simulink model "MotorDriveThermalTestbench"  (R2024b)
settings: Solver=daessc  StartTime=0.0  StopTime=2400  FixedStep=dt  RelTol=1e-3  AbsTol=1e-3
PreLoadFcn:
  | % Simulation parameters
  | MotorDriveThermalTestBenchParams;
model workspace (MAT data in the model file):
  V_frac_bridge = 0.0437
  V_fract_teeth = 0.9563
values from neighbouring files (symbols this model uses):
  CaseParams = struct()    [InverterThermalParams.m]
  HeatsinkParams = struct()    [InverterThermalParams.m]
undefined symbols (not defined in the file or in its folder): electricDrive, H_AH, H_AL, H_BH, H_BL, H_CH, H_CL, PipeParams, vehicleThermal
libraries: fl_lib x171, ee_lib x31, nesl_utility x28, nesl_utility_internal x12, sdl_lib x6, SimscapeFluids_lib x3, autolibshared x1
(part 4 of 4)

== system MotorDriveThermalTestbench/Motor Cooling/windingOilJet/ThermalResistance /Oil Wet Area ==
  PS Divide : fl_lib/Physical Signals/Functions/PS Divide
  PS Gain : fl_lib/Physical Signals/Functions/PS Gain  gain=pi
  PS Product : fl_lib/Physical Signals/Functions/PS Product
  PS Product1 : fl_lib/Physical Signals/Functions/PS Product
  Q : PMIOPort  Side=Left
  oilThickness : PMIOPort  Port=2  Side=Left
  v : PMIOPort  Port=3  Side=Left
  OD : PMIOPort  Port=4  Side=Left
  Area : PMIOPort  Port=5  Side=Right
  connections:
  Q/RConn1 -- PS Divide/LConn1
  v/RConn1 -- PS Product/LConn2
  oilThickness/RConn1 -- PS Product/LConn1
  PS Product1/RConn1 -- Area/RConn1
  PS Gain/RConn1 -- PS Product1/LConn2
  PS Product/RConn1 -- PS Divide/LConn2
  PS Divide/RConn1 -- PS Product1/LConn1
  OD/RConn1 -- PS Gain/LConn1

== system MotorDriveThermalTestbench/Motor Cooling/windingOilJet/ThermalResistance /ReynoldsNo ==
  KinamaticVisc : fl_lib/Physical Signals/Sources/PS Constant  constant=electricDrive.MotorThermal.KinVisc*1e-6 m^2/s
  PS Divide : fl_lib/Physical Signals/Functions/PS Divide
  PS Gain : fl_lib/Physical Signals/Functions/PS Gain  gain=pi
  PS Product : fl_lib/Physical Signals/Functions/PS Product
  v : PMIOPort  Side=Left
  od : PMIOPort  Port=2  Side=Left
  Re : PMIOPort  Port=3  Side=Right
  connections:
  KinamaticVisc/RConn1 -- PS Divide/LConn2
  od/RConn1 -- PS Gain/LConn1
  PS Gain/RConn1 -- PS Product/LConn2
  PS Product/RConn1 -- PS Divide/LConn1
  PS Divide/RConn1 -- Re/RConn1
  v/RConn1 -- PS Product/LConn1

== system MotorDriveThermalTestbench/Motor Cooling/windingOilJet/ThermalResistance /avgDriftVelocity ==
  "Jet Velocity " : fl_lib/Physical Signals/Sources/PS Constant  constant=0.5 m/s
  PS Add : fl_lib/Physical Signals/Functions/PS Add
  PS Add1 : fl_lib/Physical Signals/Functions/PS Add
  PS Gain : fl_lib/Physical Signals/Functions/PS Gain  gain=2*9.81 m/s^2
  PS Gain1 : fl_lib/Physical Signals/Functions/PS Gain  gain=0.5
  PS Math Function : fl_lib/Physical Signals/Functions/PS Math Function  fcn_choice=foundation.enum.math_function.square  v=1
  PS Math Function1 : fl_lib/Physical Signals/Functions/PS Math Function  fcn_choice=foundation.enum.math_function.sqrt  v=1
  vd : PMIOPort  Side=Right
  v : PMIOPort  Port=2  Side=Left
  connections:
  PS Gain/RConn1 -- PS Add/LConn2
  PS Math Function/RConn1 -- PS Add/LConn1
  PS Math Function1/RConn1 -- PS Add1/LConn2
  v/RConn1 -- PS Gain/LConn1
  "Jet Velocity "/RConn1 -- PS Math Function/LConn1 -- PS Add1/LConn1
  PS Add/RConn1 -- PS Math Function1/LConn1
  PS Gain1/LConn1 -- PS Add1/RConn1
  PS Gain1/RConn1 -- vd/RConn1

== system MotorDriveThermalTestbench/Test Env N Controls/Motor speed N test environment/Test Environment/Setting ==
  note: Road Wind & Brake
  dec : Inport
  Brake : Constant  Value=0
  Brake1 : Constant
  Bus : Subsystem
  Road Inclination : Constant  Value=0
  Switch : Switch  Criteria=u2 > Threshold  Threshold=-20.557  SaturateOnIntegerOverflow=off  InputSameDT=off
  Wind Speed : Constant  Value=0
  b : Outport
  wires:
  Bus/1(b) -> b/1
  Brake1/1 -> Switch/3
  Brake/1 -> Switch/1
  Switch/1 -> Bus/3(Br)
  dec/1 -> Switch/2
  Road Inclination/1 -> Bus/1(In)
  Wind Speed/1 -> Bus/2(Wi)

== system MotorDriveThermalTestbench/Inverter/DetailedInverter/BaseplateAndHeatsink/BasePLT/meas_AH ==
  Heat Flow Rate Sensor : fl_lib/Thermal/Thermal Sensors/Heat Flow Rate Sensor
  PS-Simulink Converter : nesl_utility_internal/PS-Simulink Converter  PhysicalDomain=network_engine_domain  SubClassName=ps_output  LeftPortType=input  RightPortType=output  PseudoPeriodic=off  Frequencies=[]  VectorFormat=inherit  Unit=degC  AffineConversion=on
  PS-Simulink Converter1 : nesl_utility_internal/PS-Simulink Converter  PhysicalDomain=network_engine_domain  SubClassName=ps_output  LeftPortType=input  RightPortType=output  PseudoPeriodic=off  Frequencies=[]  VectorFormat=inherit  Unit=W  AffineConversion=off
  Temperature Sensor : fl_lib/Thermal/Thermal Sensors/Temperature Sensor  temperature_measure=foundation.enum.MeasurementReference.difference
  Thermal Reference : fl_lib/Thermal/Thermal Elements/Thermal Reference
  A : PMIOPort  Side=Left
  B : PMIOPort  Port=2  Side=Right
  T : Outport
  Q : Outport  Port=2
  wires:
  PS-Simulink Converter/1 -> T/1
  PS-Simulink Converter1/1 -> Q/1
  connections:
  Temperature Sensor/LConn1 -- A/RConn1 -- Heat Flow Rate Sensor/LConn1
  Thermal Reference/LConn1 -- Temperature Sensor/RConn1
  PS-Simulink Converter/LConn1 -- Temperature Sensor/RConn2
  B/RConn1 -- Heat Flow Rate Sensor/RConn2
  Heat Flow Rate Sensor/RConn1 -- PS-Simulink Converter1/LConn1

== system MotorDriveThermalTestbench/Inverter/DetailedInverter/BaseplateAndHeatsink/BasePLT/meas_AL ==
  Heat Flow Rate Sensor : fl_lib/Thermal/Thermal Sensors/Heat Flow Rate Sensor
  PS-Simulink Converter : nesl_utility_internal/PS-Simulink Converter  PhysicalDomain=network_engine_domain  SubClassName=ps_output  LeftPortType=input  RightPortType=output  PseudoPeriodic=off  Frequencies=[]  VectorFormat=inherit  Unit=degC  AffineConversion=on
  PS-Simulink Converter1 : nesl_utility_internal/PS-Simulink Converter  PhysicalDomain=network_engine_domain  SubClassName=ps_output  LeftPortType=input  RightPortType=output  PseudoPeriodic=off  Frequencies=[]  VectorFormat=inherit  Unit=W  AffineConversion=off
  Temperature Sensor : fl_lib/Thermal/Thermal Sensors/Temperature Sensor  temperature_measure=foundation.enum.MeasurementReference.difference
  Thermal Reference : fl_lib/Thermal/Thermal Elements/Thermal Reference
  A : PMIOPort  Side=Left
  B : PMIOPort  Port=2  Side=Right
  T : Outport
  Q : Outport  Port=2
  wires:
  PS-Simulink Converter/1 -> T/1
  PS-Simulink Converter1/1 -> Q/1
  connections:
  Heat Flow Rate Sensor/LConn1 -- Temperature Sensor/LConn1 -- A/RConn1
  Thermal Reference/LConn1 -- Temperature Sensor/RConn1
  PS-Simulink Converter/LConn1 -- Temperature Sensor/RConn2
  B/RConn1 -- Heat Flow Rate Sensor/RConn2
  Heat Flow Rate Sensor/RConn1 -- PS-Simulink Converter1/LConn1

== system MotorDriveThermalTestbench/Inverter/DetailedInverter/BaseplateAndHeatsink/BasePLT/meas_BH ==
  Heat Flow Rate Sensor : fl_lib/Thermal/Thermal Sensors/Heat Flow Rate Sensor
  PS-Simulink Converter : nesl_utility_internal/PS-Simulink Converter  PhysicalDomain=network_engine_domain  SubClassName=ps_output  LeftPortType=input  RightPortType=output  PseudoPeriodic=off  Frequencies=[]  VectorFormat=inherit  Unit=degC  AffineConversion=on
  PS-Simulink Converter1 : nesl_utility_internal/PS-Simulink Converter  PhysicalDomain=network_engine_domain  SubClassName=ps_output  LeftPortType=input  RightPortType=output  PseudoPeriodic=off  Frequencies=[]  VectorFormat=inherit  Unit=W  AffineConversion=off
  Temperature Sensor : fl_lib/Thermal/Thermal Sensors/Temperature Sensor  temperature_measure=foundation.enum.MeasurementReference.difference
  Thermal Reference : fl_lib/Thermal/Thermal Elements/Thermal Reference
  A : PMIOPort  Side=Left
  B : PMIOPort  Port=2  Side=Right
  T : Outport
  Q : Outport  Port=2
  wires:
  PS-Simulink Converter/1 -> T/1
  PS-Simulink Converter1/1 -> Q/1
  connections:
  Heat Flow Rate Sensor/LConn1 -- Temperature Sensor/LConn1 -- A/RConn1
  Thermal Reference/LConn1 -- Temperature Sensor/RConn1
  PS-Simulink Converter/LConn1 -- Temperature Sensor/RConn2
  B/RConn1 -- Heat Flow Rate Sensor/RConn2
  Heat Flow Rate Sensor/RConn1 -- PS-Simulink Converter1/LConn1

== system MotorDriveThermalTestbench/Inverter/DetailedInverter/BaseplateAndHeatsink/BasePLT/meas_BL ==
  Heat Flow Rate Sensor : fl_lib/Thermal/Thermal Sensors/Heat Flow Rate Sensor
  PS-Simulink Converter : nesl_utility_internal/PS-Simulink Converter  PhysicalDomain=network_engine_domain  SubClassName=ps_output  LeftPortType=input  RightPortType=output  PseudoPeriodic=off  Frequencies=[]  VectorFormat=inherit  Unit=degC  AffineConversion=on
  PS-Simulink Converter1 : nesl_utility_internal/PS-Simulink Converter  PhysicalDomain=network_engine_domain  SubClassName=ps_output  LeftPortType=input  RightPortType=output  PseudoPeriodic=off  Frequencies=[]  VectorFormat=inherit  Unit=W  AffineConversion=off
  Temperature Sensor : fl_lib/Thermal/Thermal Sensors/Temperature Sensor  temperature_measure=foundation.enum.MeasurementReference.difference
  Thermal Reference : fl_lib/Thermal/Thermal Elements/Thermal Reference
  A : PMIOPort  Side=Left
  B : PMIOPort  Port=2  Side=Right
  T : Outport
  Q : Outport  Port=2
  wires:
  PS-Simulink Converter/1 -> T/1
  PS-Simulink Converter1/1 -> Q/1
  connections:
  Heat Flow Rate Sensor/LConn1 -- Temperature Sensor/LConn1 -- A/RConn1
  Thermal Reference/LConn1 -- Temperature Sensor/RConn1
  PS-Simulink Converter/LConn1 -- Temperature Sensor/RConn2
  B/RConn1 -- Heat Flow Rate Sensor/RConn2
  Heat Flow Rate Sensor/RConn1 -- PS-Simulink Converter1/LConn1

== system MotorDriveThermalTestbench/Inverter/DetailedInverter/BaseplateAndHeatsink/BasePLT/meas_CH ==
  Heat Flow Rate Sensor : fl_lib/Thermal/Thermal Sensors/Heat Flow Rate Sensor
  PS-Simulink Converter : nesl_utility_internal/PS-Simulink Converter  PhysicalDomain=network_engine_domain  SubClassName=ps_output  LeftPortType=input  RightPortType=output  PseudoPeriodic=off  Frequencies=[]  VectorFormat=inherit  Unit=degC  AffineConversion=on
  PS-Simulink Converter1 : nesl_utility_internal/PS-Simulink Converter  PhysicalDomain=network_engine_domain  SubClassName=ps_output  LeftPortType=input  RightPortType=output  PseudoPeriodic=off  Frequencies=[]  VectorFormat=inherit  Unit=W  AffineConversion=off
  Temperature Sensor : fl_lib/Thermal/Thermal Sensors/Temperature Sensor  temperature_measure=foundation.enum.MeasurementReference.difference
  Thermal Reference : fl_lib/Thermal/Thermal Elements/Thermal Reference
  A : PMIOPort  Side=Left
  B : PMIOPort  Port=2  Side=Right
  T : Outport
  Q : Outport  Port=2
  wires:
  PS-Simulink Converter/1 -> T/1
  PS-Simulink Converter1/1 -> Q/1
  connections:
  Heat Flow Rate Sensor/LConn1 -- Temperature Sensor/LConn1 -- A/RConn1
  Thermal Reference/LConn1 -- Temperature Sensor/RConn1
  PS-Simulink Converter/LConn1 -- Temperature Sensor/RConn2
  B/RConn1 -- Heat Flow Rate Sensor/RConn2
  Heat Flow Rate Sensor/RConn1 -- PS-Simulink Converter1/LConn1

== system MotorDriveThermalTestbench/Inverter/DetailedInverter/BaseplateAndHeatsink/BasePLT/meas_CL ==
  Heat Flow Rate Sensor : fl_lib/Thermal/Thermal Sensors/Heat Flow Rate Sensor
  PS-Simulink Converter : nesl_utility_internal/PS-Simulink Converter  PhysicalDomain=network_engine_domain  SubClassName=ps_output  LeftPortType=input  RightPortType=output  PseudoPeriodic=off  Frequencies=[]  VectorFormat=inherit  Unit=degC  AffineConversion=on
  PS-Simulink Converter1 : nesl_utility_internal/PS-Simulink Converter  PhysicalDomain=network_engine_domain  SubClassName=ps_output  LeftPortType=input  RightPortType=output  PseudoPeriodic=off  Frequencies=[]  VectorFormat=inherit  Unit=W  AffineConversion=off
  Temperature Sensor : fl_lib/Thermal/Thermal Sensors/Temperature Sensor  temperature_measure=foundation.enum.MeasurementReference.difference
  Thermal Reference : fl_lib/Thermal/Thermal Elements/Thermal Reference
  A : PMIOPort  Side=Left
  B : PMIOPort  Port=2  Side=Right
  T : Outport
  Q : Outport  Port=2
  wires:
  PS-Simulink Converter/1 -> T/1
  PS-Simulink Converter1/1 -> Q/1
  connections:
  Heat Flow Rate Sensor/LConn1 -- Temperature Sensor/LConn1 -- A/RConn1
  Thermal Reference/LConn1 -- Temperature Sensor/RConn1
  PS-Simulink Converter/LConn1 -- Temperature Sensor/RConn2
  B/RConn1 -- Heat Flow Rate Sensor/RConn2
  Heat Flow Rate Sensor/RConn1 -- PS-Simulink Converter1/LConn1

== system MotorDriveThermalTestbench/Inverter/DetailedInverter/BaseplateAndHeatsink/HeatSink/HeatConduction ==
  Heatsink1 : ee_lib/Passive/Thermal/Heatsink  parameterization=ee.enum.passive.thermal.heatsinkParam.rectangularFin  convection=ee.enum.passive.thermal.heatsinkConvection.specifyFlowSpeed  T_vec_Q=[10, 30, 50, 70, 90] K  v_vec_Q=[0, 1, 2, 3] m/s  Q_TLU1=[6.1, 23.6, 44.5, 67.5, 92.3] W  Q_TLU2=[6.1, 18.8, 22.8, 25.7; 23.6, 61.1, 73, 81.5; 44.5, 106.4, 125.9, 140.1; 67.5, 153.5, 180.7, 200.3; 92.3, 202.1, 236.9, 262] W  T_vec_h=[10, 30, 50, 70, 90] K  v_vec_h=[0, 1, 2, 3] m/s  h_TLU1=[5.4, 7.02, 7.98, 8.68, 9.26] W/(K*m^2)  h_TLU2=[5.4, 17.86, 22.17, 25.41; 7.02, 19.49, 23.8, 27.03; 7.97, 20.44, 24.75, 27.99; 8.68, 21.15, 25.46, 28.69; 9.26, 21.73, 26.04, 29.27] W/(K*m^2)  h_vec=[5, 10, 15, 20, 25, 30] W/(K*m^2)  eff_TLU=[96.97, 94.16, 91.53, 89.08, 86.78, 84.62]  height=HeatsinkParams.Height m  thick=HeatsinkParams.Thick m  depth=HeatsinkParams.Depth m  gap=HeatsinkParams.Gap m  num_fins=HeatsinkParams.NumFins/3  k_fin=386 W/(K*m)  A_total=0.1171 m^2  nu=2.62e-6 m^2/s  alpha=6.55e-8 m^2/s  k_fluid=0.55 W/(K*m)  beta=5.82e-4 1/K  mass=HeatsinkParams.Mass kg  sp_heat=437 J/(K*kg)  T_hs_specify=on  T_hs_priority=High  T_hs=Tamb degC  T_hs_nominal_specify=off  T_hs_nominal_value=1  T_hs_nominal_unit=K  Q_A_specify=off  Q_A_priority=None  Q_A=0 W  Q_A_nominal_specify=on  Q_A_nominal_value=1  Q_A_nominal_unit=W  Q_C_specify=off  Q_C_priority=None  Q_C=0 W  Q_C_nominal_specify=on  Q_C_nominal_value=1  Q_C_nominal_unit=W
      settings: InternalSimscapePortConfiguration="{\"Bottom\":[{\"id\":\"C\",\"label\":\"C\",\"type\":\"foundation.thermal.thermal\"}],\"Left\":[{\"id\":\"v\",\"label\":\"v\",\"type\":\"input\"}],\"Right\":[],\"Top\":[{\"id\":\"A\",\"label\":\"A\",\"type\":\"foundation.thermal.thermal\"}]}"
  Heatsink2 : ee_lib/Passive/Thermal/Heatsink  parameterization=ee.enum.passive.thermal.heatsinkParam.rectangularFin  convection=ee.enum.passive.thermal.heatsinkConvection.specifyFlowSpeed  T_vec_Q=[10, 30, 50, 70, 90] K  v_vec_Q=[0, 1, 2, 3] m/s  Q_TLU1=[6.1, 23.6, 44.5, 67.5, 92.3] W  Q_TLU2=[6.1, 18.8, 22.8, 25.7; 23.6, 61.1, 73, 81.5; 44.5, 106.4, 125.9, 140.1; 67.5, 153.5, 180.7, 200.3; 92.3, 202.1, 236.9, 262] W  T_vec_h=[10, 30, 50, 70, 90] K  v_vec_h=[0, 1, 2, 3] m/s  h_TLU1=[5.4, 7.02, 7.98, 8.68, 9.26] W/(K*m^2)  h_TLU2=[5.4, 17.86, 22.17, 25.41; 7.02, 19.49, 23.8, 27.03; 7.97, 20.44, 24.75, 27.99; 8.68, 21.15, 25.46, 28.69; 9.26, 21.73, 26.04, 29.27] W/(K*m^2)  h_vec=[5, 10, 15, 20, 25, 30] W/(K*m^2)  eff_TLU=[96.97, 94.16, 91.53, 89.08, 86.78, 84.62]  height=HeatsinkParams.Height m  thick=HeatsinkParams.Thick m  depth=HeatsinkParams.Depth m  gap=HeatsinkParams.Gap m  num_fins=HeatsinkParams.NumFins/3  k_fin=386 W/(K*m)  A_total=0.1171 m^2  nu=2.62e-6 m^2/s  alpha=6.55e-8 m^2/s  k_fluid=0.55 W/(K*m)  beta=5.82e-4 1/K  mass=HeatsinkParams.Mass kg  sp_heat=437 J/(K*kg)  T_hs_specify=on  T_hs_priority=High  T_hs=Tamb degC  T_hs_nominal_specify=off  T_hs_nominal_value=1  T_hs_nominal_unit=K  Q_A_specify=off  Q_A_priority=None  Q_A=0 W  Q_A_nominal_specify=on  Q_A_nominal_value=1  Q_A_nominal_unit=W  Q_C_specify=off  Q_C_priority=None  Q_C=0 W  Q_C_nominal_specify=on  Q_C_nominal_value=1  Q_C_nominal_unit=W
      settings: InternalSimscapePortConfiguration="{\"Bottom\":[{\"id\":\"C\",\"label\":\"C\",\"type\":\"foundation.thermal.thermal\"}],\"Left\":[{\"id\":\"v\",\"label\":\"v\",\"type\":\"input\"}],\"Right\":[],\"Top\":[{\"id\":\"A\",\"label\":\"A\",\"type\":\"foundation.thermal.thermal\"}]}"
  Heatsink3 : ee_lib/Passive/Thermal/Heatsink  parameterization=ee.enum.passive.thermal.heatsinkParam.rectangularFin  convection=ee.enum.passive.thermal.heatsinkConvection.specifyFlowSpeed  T_vec_Q=[10, 30, 50, 70, 90] K  v_vec_Q=[0, 1, 2, 3] m/s  Q_TLU1=[6.1, 23.6, 44.5, 67.5, 92.3] W  Q_TLU2=[6.1, 18.8, 22.8, 25.7; 23.6, 61.1, 73, 81.5; 44.5, 106.4, 125.9, 140.1; 67.5, 153.5, 180.7, 200.3; 92.3, 202.1, 236.9, 262] W  T_vec_h=[10, 30, 50, 70, 90] K  v_vec_h=[0, 1, 2, 3] m/s  h_TLU1=[5.4, 7.02, 7.98, 8.68, 9.26] W/(K*m^2)  h_TLU2=[5.4, 17.86, 22.17, 25.41; 7.02, 19.49, 23.8, 27.03; 7.97, 20.44, 24.75, 27.99; 8.68, 21.15, 25.46, 28.69; 9.26, 21.73, 26.04, 29.27] W/(K*m^2)  h_vec=[5, 10, 15, 20, 25, 30] W/(K*m^2)  eff_TLU=[96.97, 94.16, 91.53, 89.08, 86.78, 84.62]  height=HeatsinkParams.Height m  thick=HeatsinkParams.Thick m  depth=HeatsinkParams.Depth m  gap=HeatsinkParams.Gap m  num_fins=HeatsinkParams.NumFins/3  k_fin=386 W/(K*m)  A_total=0.1171 m^2  nu=2.62e-6 m^2/s  alpha=6.55e-8 m^2/s  k_fluid=0.55 W/(K*m)  beta=5.82e-4 1/K  mass=HeatsinkParams.Mass kg  sp_heat=437 J/(K*kg)  T_hs_specify=on  T_hs_priority=High  T_hs=Tamb degC  T_hs_nominal_specify=off  T_hs_nominal_value=1  T_hs_nominal_unit=K  Q_A_specify=off  Q_A_priority=None  Q_A=0 W  Q_A_nominal_specify=on  Q_A_nominal_value=1  Q_A_nominal_unit=W  Q_C_specify=off  Q_C_priority=None  Q_C=0 W  Q_C_nominal_specify=on  Q_C_nominal_value=1  Q_C_nominal_unit=W
      settings: InternalSimscapePortConfiguration="{\"Bottom\":[{\"id\":\"C\",\"label\":\"C\",\"type\":\"foundation.thermal.thermal\"}],\"Left\":[{\"id\":\"v\",\"label\":\"v\",\"type\":\"input\"}],\"Right\":[],\"Top\":[{\"id\":\"A\",\"label\":\"A\",\"type\":\"foundation.thermal.thermal\"}]}"
  coolantV : PMIOPort  Side=Left
  Ha : PMIOPort  Port=2  Side=Right
  Hb : PMIOPort  Port=3  Side=Right
  Hc : PMIOPort  Port=4  Side=Right
  " " : PMIOPort  Port=5  Side=Left
  "  " : PMIOPort  Port=6  Side=Left
  "   " : PMIOPort  Port=7  Side=Left
  connections:
  Heatsink3/LConn1 -- Heatsink1/LConn1 -- coolantV/RConn1 -- Heatsink2/LConn1
  Hb/RConn1 -- Heatsink2/LConn2
  Hc/RConn1 -- Heatsink1/LConn2
  "  "/RConn1 -- Heatsink2/RConn1
  " "/RConn1 -- Heatsink3/RConn1
  Ha/RConn1 -- Heatsink3/LConn2
  "   "/RConn1 -- Heatsink1/RConn1

== system MotorDriveThermalTestbench/Inverter/DetailedInverter/BaseplateAndHeatsink/HeatSink/HeatConvection ==
  HS Eq Pipe : fl_lib/Thermal Liquid/Elements/Pipe (TL)  length=1.1*HeatsinkParams.ChennelLength/3 m  area=HeatsinkParams.EqPipeDia^2*pi/4 m^2  Dh=HeatsinkParams.EqPipeDia m  length_add=HeatsinkParams.EqLengthRough m  roughness=HeatsinkParams.EqPipeRoughness m  Re_lam=2000  Re_tur=4000  shape_factor=64  Nu_lam=3000  dynamic_compressibility=simscape.enum.onoff.off  inertia=simscape.enum.onoff.off  p0=0.101325 MPa  T0=Tamb degC  mdot0=0 kg/s
  HS Eq Pipe1 : fl_lib/Thermal Liquid/Elements/Pipe (TL)  length=1.1*HeatsinkParams.ChennelLength/3 m  area=HeatsinkParams.EqPipeDia^2*pi/4 m^2  Dh=HeatsinkParams.EqPipeDia m  length_add=HeatsinkParams.EqLengthRough m  roughness=HeatsinkParams.EqPipeRoughness m  Re_lam=2000  Re_tur=4000  shape_factor=64  Nu_lam=3000  dynamic_compressibility=simscape.enum.onoff.off  inertia=simscape.enum.onoff.off  p0=0.101325 MPa  T0=Tamb degC  mdot0=0 kg/s
  HS Eq Pipe2 : fl_lib/Thermal Liquid/Elements/Pipe (TL)  length=1.1*HeatsinkParams.ChennelLength/3 m  area=HeatsinkParams.EqPipeDia^2*pi/4 m^2  Dh=HeatsinkParams.EqPipeDia m  length_add=HeatsinkParams.EqLengthRough m  roughness=HeatsinkParams.EqPipeRoughness m  Re_lam=2000  Re_tur=4000  shape_factor=64  Nu_lam=3000  dynamic_compressibility=simscape.enum.onoff.off  inertia=simscape.enum.onoff.off  p0=0.101325 MPa  T0=Tamb degC  mdot0=0 kg/s
  coolantIn : PMIOPort  Side=Left
  coolantOut : PMIOPort  Port=2  Side=Right
  Ha : PMIOPort  Port=3  Side=Left
  Hb : PMIOPort  Port=4  Side=Left
  Hc : PMIOPort  Port=5  Side=Left
  connections:
  HS Eq Pipe1/RConn1 -- HS Eq Pipe/LConn1
  HS Eq Pipe2/RConn1 -- HS Eq Pipe1/LConn1
  HS Eq Pipe1/LConn2 -- Hb/RConn1
  HS Eq Pipe/LConn2 -- Ha/RConn1
  HS Eq Pipe2/LConn2 -- Hc/RConn1
  HS Eq Pipe2/LConn1 -- coolantOut/RConn1
  HS Eq Pipe/RConn1 -- coolantIn/RConn1

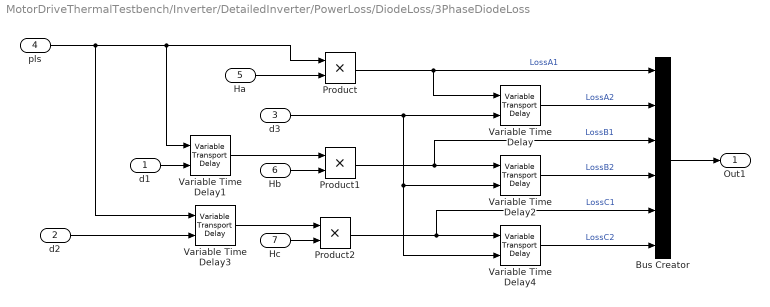
== system MotorDriveThermalTestbench/Inverter/DetailedInverter/PowerLoss/DiodeLoss/3PhaseDiodeLoss ==
  d1 : Inport
  d2 : Inport  Port=2
  d3 : Inport  Port=3
  pls : Inport  Port=4
  Ha : Inport  Port=5
  Hb : Inport  Port=6
  Hc : Inport  Port=7
  Bus Creator : BusCreator  Inputs=6
  Product : Product
  Product1 : Product
  Product2 : Product
  Variable Time Delay{,1..4} (5 alike) : VariableTransportDelay  VariableDelayType=Variable transport delay  MaximumDelay=60  MaximumPoints=75000  TransDelayFeedthrough=on
  Out1 : Outport
  wires:
  Product2/1 -> Variable Time Delay4/1, Bus Creator/5  "LossC1"
  Product/1 -> Variable Time Delay/1, Bus Creator/1  "LossA1"
  Bus Creator/1 -> Out1/1
  Variable Time Delay3/1 -> Product2/1
  Product1/1 -> Bus Creator/3, Variable Time Delay2/1  "LossB1"
  Variable Time Delay/1 -> Bus Creator/2  "LossA2"
  Variable Time Delay1/1 -> Product1/1
  Variable Time Delay4/1 -> Bus Creator/6  "LossC2"
  Variable Time Delay2/1 -> Bus Creator/4  "LossB2"
  d2/1 -> Variable Time Delay3/2
  Ha/1 -> Product/2
  d1/1 -> Variable Time Delay1/2
  Hb/1 -> Product1/2
  Hc/1 -> Product2/2
  d3/1 -> Variable Time Delay4/2, Variable Time Delay2/2, Variable Time Delay/2
  pls/1 -> Variable Time Delay3/1, Product/1, Variable Time Delay1/1

== system MotorDriveThermalTestbench/Inverter/DetailedInverter/PowerLoss/DiodeLoss/DiodeLossTbl ==
  momega : Inport
  mtq : Inport  Port=2
  temp : Inport  Port=3
  Abs : Abs  SaturateOnIntegerOverflow=off
  Bus Selector : BusSelector  OutputSignals=TdA,TdB,TdC
  LossTables1 : Subsystem
  Transfer Fcn : TransferFcn  Denominator=[0.1 1]
  Transfer Fcn1 : TransferFcn  Denominator=[0.1 1]
  Transfer Fcn2 : TransferFcn  Denominator=[0.1 1]
  Ha : Outport
  Hb : Outport  Port=2
  Hc : Outport  Port=3
  wires:
  Transfer Fcn/1 -> LossTables1/3(T1)
  momega/1 -> LossTables1/1(w)
  Transfer Fcn1/1 -> LossTables1/4(T2)
  Abs/1 -> LossTables1/2(tq)
  Bus Selector/2 -> Transfer Fcn1/1  "<TdB>"
  Bus Selector/1 -> Transfer Fcn/1  "<TdA>"
  Transfer Fcn2/1 -> LossTables1/5(T3)
  Bus Selector/3 -> Transfer Fcn2/1  "<TdC>"
  LossTables1/1(H1) -> Ha/1
  LossTables1/2(H2) -> Hb/1
  LossTables1/3(H3) -> Hc/1
  temp/1 -> Bus Selector/1
  mtq/1 -> Abs/1

== system MotorDriveThermalTestbench/Inverter/DetailedInverter/PowerLoss/DiodeLoss/DutyCycle ==
  motRPM : Inport
  Abs : Abs  SaturateOnIntegerOverflow=off
  Constant2 : Constant  Value=3
  Constant3 : Constant
  Divide1 : Product  Inputs=*/
  Gain : Gain  Gain=2
  Gain1 : Gain  Gain=1.5
  Math Function1 : Math  Operator=reciprocal
  Sum : Sum  Inputs=|++
  SynchroHz : Gain  Gain=0.3*electricDrive.MotorThermal.Npl/60
  Transfer Fcn : TransferFcn  Denominator=[0.1 1]
  d1 : Outport
  d2 : Outport  Port=2
  d3 : Outport  Port=3
  timeperiod : Outport  Port=4
  MotOmega : Outport  Port=5
  wires:
  Constant2/1 -> Divide1/2
  Divide1/1 -> d1/1, Gain/1, Gain1/1
  Gain1/1 -> d3/1
  Constant3/1 -> Sum/2
  motRPM/1 -> Transfer Fcn/1
  Gain/1 -> d2/1
  Abs/1 -> Sum/1, MotOmega/1
  Sum/1 -> SynchroHz/1
  Transfer Fcn/1 -> Abs/1
  Math Function1/1 -> timeperiod/1, Divide1/1
  SynchroHz/1 -> Math Function1/1

== system MotorDriveThermalTestbench/Inverter/DetailedInverter/PowerLoss/DiodeLoss/VariablePulse ==
  ds : Inport
  timeperiod : Inport  Port=2
  Math Function : Math  Operator=reciprocal
  Product : Product
  Variable Pulse Generator : VariablePulseGenerator  SampleTime=0.1
  pulse : Outport
  wires:
  timeperiod/1 -> Variable Pulse Generator/2
  ds/1 -> Math Function/1, Variable Pulse Generator/1
  Variable Pulse Generator/1 -> Product/2
  Math Function/1 -> Product/1
  Product/1 -> pulse/1

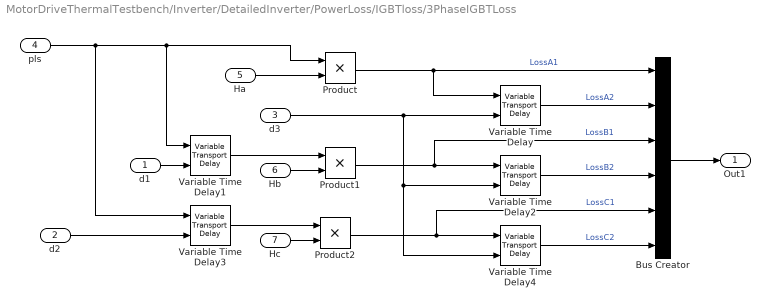
== system MotorDriveThermalTestbench/Inverter/DetailedInverter/PowerLoss/IGBTloss/3PhaseIGBTLoss ==
  d1 : Inport
  d2 : Inport  Port=2
  d3 : Inport  Port=3
  pls : Inport  Port=4
  Ha : Inport  Port=5
  Hb : Inport  Port=6
  Hc : Inport  Port=7
  Bus Creator : BusCreator  Inputs=6
  Product : Product
  Product1 : Product
  Product2 : Product
  Variable Time Delay{,1..4} (5 alike) : VariableTransportDelay  VariableDelayType=Variable transport delay  MaximumDelay=60  MaximumPoints=75000  TransDelayFeedthrough=on
  Out1 : Outport
  wires:
  Product2/1 -> Variable Time Delay4/1, Bus Creator/5  "LossC1"
  Product/1 -> Variable Time Delay/1, Bus Creator/1  "LossA1"
  Bus Creator/1 -> Out1/1
  Variable Time Delay3/1 -> Product2/1
  Product1/1 -> Bus Creator/3, Variable Time Delay2/1  "LossB1"
  Variable Time Delay/1 -> Bus Creator/2  "LossA2"
  Variable Time Delay1/1 -> Product1/1
  Variable Time Delay4/1 -> Bus Creator/6  "LossC2"
  Variable Time Delay2/1 -> Bus Creator/4  "LossB2"
  d2/1 -> Variable Time Delay3/2
  Ha/1 -> Product/2
  d1/1 -> Variable Time Delay1/2
  Hb/1 -> Product1/2
  Hc/1 -> Product2/2
  d3/1 -> Variable Time Delay4/2, Variable Time Delay2/2, Variable Time Delay/2
  pls/1 -> Variable Time Delay3/1, Product/1, Variable Time Delay1/1

== system MotorDriveThermalTestbench/Inverter/DetailedInverter/PowerLoss/IGBTloss/DutyCycle ==
  motRPM : Inport
  Abs : Abs  SaturateOnIntegerOverflow=off
  Constant2 : Constant  Value=3
  Constant3 : Constant
  Divide1 : Product  Inputs=*/
  Gain : Gain  Gain=2
  Gain1 : Gain  Gain=1.5
  Math Function : Math  Operator=reciprocal
  Sum : Sum  Inputs=|++
  SynchroHz/3 : Gain  Gain=0.3*electricDrive.MotorThermal.Npl/60
  Transfer Fcn : TransferFcn  Denominator=[0.1 1]
  d1 : Outport
  d2 : Outport  Port=2
  d3 : Outport  Port=3
  timeperiod : Outport  Port=4
  MotOmega : Outport  Port=5
  wires:
  Constant2/1 -> Divide1/2
  Divide1/1 -> Gain1/1, d1/1, Gain/1
  Gain1/1 -> d3/1
  Constant3/1 -> Sum/2
  motRPM/1 -> Transfer Fcn/1
  Gain/1 -> d2/1
  SynchroHz/3/1 -> Math Function/1
  Sum/1 -> SynchroHz/3/1, MotOmega/1
  Abs/1 -> Sum/1
  Transfer Fcn/1 -> Abs/1
  Math Function/1 -> Divide1/1, timeperiod/1

== system MotorDriveThermalTestbench/Inverter/DetailedInverter/PowerLoss/IGBTloss/IGBTLossTbl ==
  momega : Inport
  mtq : Inport  Port=2
  temp : Inport  Port=3
  Abs : Abs  SaturateOnIntegerOverflow=off
  Bus Selector : BusSelector  OutputSignals=TiA,TiB,TiC
  LossTables1 : Subsystem
  Transfer Fcn : TransferFcn  Denominator=[0.1 1]
  Transfer Fcn1 : TransferFcn  Denominator=[0.1 1]
  Transfer Fcn2 : TransferFcn  Denominator=[0.1 1]
  Ha : Outport
  Hb : Outport  Port=2
  Hc : Outport  Port=3
  wires:
  Transfer Fcn/1 -> LossTables1/3(T1)
  momega/1 -> LossTables1/1(w)
  Transfer Fcn1/1 -> LossTables1/4(T2)
  Abs/1 -> LossTables1/2(tq)
  Bus Selector/2 -> Transfer Fcn1/1  "<TiB>"
  Bus Selector/1 -> Transfer Fcn/1  "<TiA>"
  Transfer Fcn2/1 -> LossTables1/5(T3)
  Bus Selector/3 -> Transfer Fcn2/1  "<TiC>"
  LossTables1/1(H1) -> Ha/1
  LossTables1/2(H2) -> Hb/1
  LossTables1/3(H3) -> Hc/1
  temp/1 -> Bus Selector/1
  mtq/1 -> Abs/1

== system MotorDriveThermalTestbench/Inverter/DetailedInverter/PowerLoss/IGBTloss/VariablePulse ==
  ds : Inport
  timeperiod : Inport  Port=2
  Math Function : Math  Operator=reciprocal
  Product : Product
  Variable Pulse Generator : VariablePulseGenerator  SampleTime=0.1
  pulse : Outport
  wires:
  Variable Pulse Generator/1 -> Product/2
  timeperiod/1 -> Variable Pulse Generator/2
  ds/1 -> Math Function/1, Variable Pulse Generator/1
  Math Function/1 -> Product/1
  Product/1 -> pulse/1

== system MotorDriveThermalTestbench/Test Env N Controls/Motor speed N test environment/Test Environment/Setting/Bus ==
  In : Inport
  Wi : Inport  Port=2
  Br : Inport  Port=3
  Bus Creator : BusCreator  Inputs=3
  b : Outport  VectorParamsAs1DForOutWhenUnconnected=off
  wires:
  Wi/1 -> Bus Creator/2  "Wind speed"
  Bus Creator/1 -> b/1
  Br/1 -> Bus Creator/3  "Brake pedal"
  In/1 -> Bus Creator/1  "Incline"

== system MotorDriveThermalTestbench/Inverter/DetailedInverter/PowerLoss/DiodeLoss/DiodeLossTbl/LossTables1 ==
  w : Inport
  tq : Inport  Port=2
  T1 : Inport  Port=3
  T2 : Inport  Port=4
  T3 : Inport  Port=5
  n-D Lookup Table1 : Lookup_n-D  NumberOfTableDimensions=3  BreakpointsForDimension1=electricDrive.motor_loss_map.spMat  BreakpointsForDimension2=electricDrive.motor_loss_map.tqMat  BreakpointsForDimension3=[298.15,398.15,448.15]  Table=electricDrive.inverter_loss_map.lossMatDiode  InternalRulePriority=Speed  RndMeth=Simplest
      settings: InputPortMap=u0,u1,u2
  n-D Lookup Table2 : Lookup_n-D  NumberOfTableDimensions=3  BreakpointsForDimension1=electricDrive.motor_loss_map.spMat  BreakpointsForDimension2=electricDrive.motor_loss_map.tqMat  BreakpointsForDimension3=[298.15,398.15,448.15]  Table=electricDrive.inverter_loss_map.lossMatDiode  InternalRulePriority=Speed  RndMeth=Simplest
      settings: InputPortMap=u0,u1,u2
  n-D Lookup Table3 : Lookup_n-D  NumberOfTableDimensions=3  BreakpointsForDimension1=electricDrive.motor_loss_map.spMat  BreakpointsForDimension2=electricDrive.motor_loss_map.tqMat  BreakpointsForDimension3=[298.15,398.15,448.15]  Table=electricDrive.inverter_loss_map.lossMatDiode  InternalRulePriority=Speed  RndMeth=Simplest
      settings: InputPortMap=u0,u1,u2
  H1 : Outport
  H2 : Outport  Port=2
  H3 : Outport  Port=3
  wires:
  T2/1 -> n-D Lookup Table3/3
  n-D Lookup Table1/1 -> H3/1
  n-D Lookup Table2/1 -> H1/1
  n-D Lookup Table3/1 -> H2/1
  w/1 -> n-D Lookup Table2/1, n-D Lookup Table1/1, n-D Lookup Table3/1
  T1/1 -> n-D Lookup Table2/3
  T3/1 -> n-D Lookup Table1/3
  tq/1 -> n-D Lookup Table2/2, n-D Lookup Table1/2, n-D Lookup Table3/2

== system MotorDriveThermalTestbench/Inverter/DetailedInverter/PowerLoss/IGBTloss/IGBTLossTbl/LossTables1 ==
  w : Inport
  tq : Inport  Port=2
  T1 : Inport  Port=3
  T2 : Inport  Port=4
  T3 : Inport  Port=5
  n-D Lookup Table : Lookup_n-D  NumberOfTableDimensions=3  BreakpointsForDimension1=electricDrive.motor_loss_map.spMat  BreakpointsForDimension2=electricDrive.motor_loss_map.tqMat  BreakpointsForDimension3=[298.15,398.15,448.15]  Table=electricDrive.inverter_loss_map.lossMatIgbt  InternalRulePriority=Speed  RndMeth=Simplest
      settings: InputPortMap=u0,u1,u2
  n-D Lookup Table1 : Lookup_n-D  NumberOfTableDimensions=3  BreakpointsForDimension1=electricDrive.motor_loss_map.spMat  BreakpointsForDimension2=electricDrive.motor_loss_map.tqMat  BreakpointsForDimension3=[298.15,398.15,448.15]  Table=electricDrive.inverter_loss_map.lossMatIgbt  InternalRulePriority=Speed  RndMeth=Simplest
      settings: InputPortMap=u0,u1,u2
  n-D Lookup Table3 : Lookup_n-D  NumberOfTableDimensions=3  BreakpointsForDimension1=electricDrive.motor_loss_map.spMat  BreakpointsForDimension2=electricDrive.motor_loss_map.tqMat  BreakpointsForDimension3=[298.15,398.15,448.15]  Table=electricDrive.inverter_loss_map.lossMatIgbt  InternalRulePriority=Speed  RndMeth=Simplest
      settings: InputPortMap=u0,u1,u2
  H1 : Outport
  H2 : Outport  Port=2
  H3 : Outport  Port=3
  wires:
  T2/1 -> n-D Lookup Table3/3
  n-D Lookup Table1/1 -> H3/1
  n-D Lookup Table/1 -> H1/1
  n-D Lookup Table3/1 -> H2/1
  w/1 -> n-D Lookup Table1/1, n-D Lookup Table3/1, n-D Lookup Table/1
  T1/1 -> n-D Lookup Table/3
  T3/1 -> n-D Lookup Table1/3
  tq/1 -> n-D Lookup Table/2, n-D Lookup Table1/2, n-D Lookup Table3/2
